simulink model "dropmodel"  (Simulink 8.7)
settings: Solver=ode23  StartTime=0.0  StopTime=3  RelTol=1e-3
undefined symbols (not defined in the file or in its folder): du0, p, u0
libraries: simulink x3
settings Model: Creator=Veikko Sariola  LastModifiedBy=sariola
settings DataIOCC: LimitDataPoints=off  SignalLoggingSaveFormat=ModelDataLogs
settings OptimizationCC: ExpressionDepthLimit=2147483647  InitFltsAndDblsToZero=on
settings DebuggingCC: SolverPrmCheckMsg=warning  FcnCallInpInsideContextMsg=UseLocalSettings  StateNameClashWarn=warning
settings GRTTargetCC: GeneratePreprocessorConditionals=Use local settings  CombineOutputUpdateFcns=off  GRTInterface=on

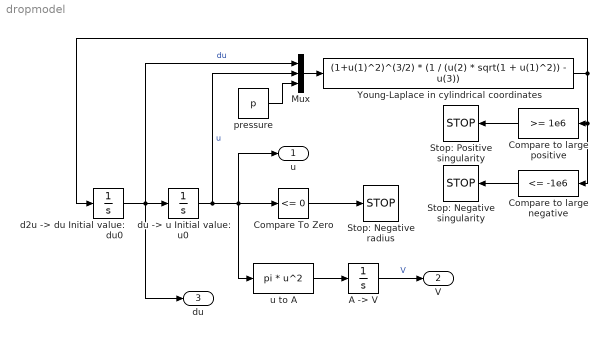
== system dropmodel ==
  "A -> V" : Integrator
  Compare To Zero : simulink/Logic and Bit Operations/Compare To Zero  relop=<=  OutDataTypeStr=boolean
  Compare to large negative : simulink/Logic and Bit Operations/Compare To Constant  relop=<=  const=-1e6  OutDataTypeStr=boolean
  "Compare to large positive " : simulink/Logic and Bit Operations/Compare To Constant  relop=>=  const=1e6  OutDataTypeStr=boolean
  Mux : Mux  Inputs=3
  Stop: Negative radius : Stop
  Stop: Negative singularity : Stop
  Stop: Positive singularity : Stop
  "Young-Laplace in cylindrical coordinates " : Fcn  Expr=(1+u(1)^2)^(3/2) * (1 / (u(2) * sqrt(1 + u(1)^2)) - u(3))
  "d2u -> du Initial value: du0" : Integrator  InitialCondition=du0
  "du -> u Initial value: u0" : Integrator  InitialCondition=u0
  pressure : Constant  Value=p
  u to A : Fcn  Expr=pi * u^2
  u : Outport
  V : Outport  Port=2
  du : Outport  Port=3
  wires:
  "d2u -> du Initial value: du0"/1 -> Mux/1, "du -> u Initial value: u0"/1, du/1  "du"
  "du -> u Initial value: u0"/1 -> Mux/2, Compare To Zero/1, u to A/1, u/1  "u"
  Compare To Zero/1 -> Stop: Negative radius/1
  u to A/1 -> "A -> V"/1
  "A -> V"/1 -> V/1  "V"
  pressure/1 -> Mux/3
  Mux/1 -> "Young-Laplace in cylindrical coordinates "/1
  "Young-Laplace in cylindrical coordinates "/1 -> Compare to large negative/1, "Compare to large positive "/1, "d2u -> du Initial value: du0"/1
  "Compare to large positive "/1 -> Stop: Positive singularity/1
  Compare to large negative/1 -> Stop: Negative singularity/1
